simulink model "boolCheck"  (R2022b)
settings: Solver=VariableStepAuto  StartTime=0.0  StopTime=10.0  RelTol=1e-3
settings Model: Creator=ChrisGeorge  LastModifiedBy=ChrisGeorge

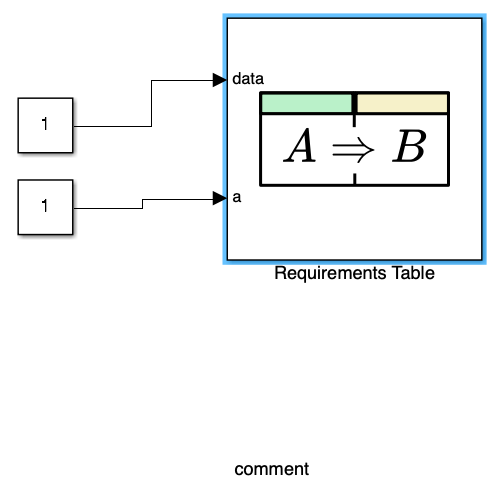
[thumbnail: Simulink's stored preview of the top-level diagram]
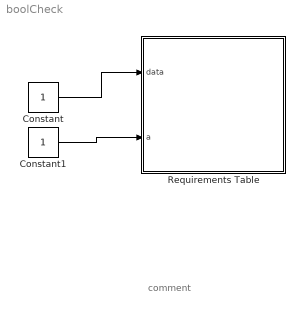
== system boolCheck ==
  note: comment
  Constant : Constant
  Constant1 : Constant
  Requirements Table : Requirements Table  TreatAsAtomicUnit=on
  wires:
  Constant/1 -> Requirements Table/1(data)
  Constant1/1 -> Requirements Table/2(a)

== stateflow chart boolCheck/Requirements Table ==
  (default) -> (junction 1073741860)
  (junction 1073741860) -> (junction 1073741861) : {
      | % SF_REQ_REV_07
      | }
  (junction 1073741861) -> (junction 1073741863) : {
      | % HEADER_ASSIGNMENTS
      |
      | }
  (junction 1073741863) -> (junction 1073741865) : {
      | % START_A_4
      | }
  (junction 1073741865) -> (junction 1073741867) : {
      | }
  (junction 1073741867) -> (junction 1073741869)
  (junction 1073741869) -> (junction 1073741871) : {
      | }
  (junction 1073741871) -> (junction 1073741873) : {
      | % END_A_4
      | }
  (junction 1073741873) -> (junction 1073741911) : {
      | % START_R_1
      | }
  (junction 1073741911) -> (junction 1073741913) : {
      | }
  (junction 1073741913) -> (junction 1073741915)
  (junction 1073741915) -> (junction 1073741917) [order 1] : [((data < 10) | (data > 10) & (data  > 10))]
  (junction 1073741915) -> (junction 1073741923) [order 2]
  (junction 1073741917) -> (junction 1073741919) : {
      | reqtable_postcondition((a > 0), 'R:1');
      |
      |
      | }
  (junction 1073741919) -> (junction 1073741921) : {
      | }
  (junction 1073741921) -> (junction 1073741923)
  (junction 1073741923) -> (junction 1073741925)
  (junction 1073741925) -> (junction 1073741927) : {
      | % END_R_1
      | }
  (junction 1073741927) -> (junction 1073741945) : {
      | % START_R_7
      | }
  (junction 1073741945) -> (junction 1073741947) : {
      | }
  (junction 1073741947) -> (junction 1073741949)
  (junction 1073741949) -> (junction 1073741951) [order 1] : [((data < 10) | (data > 10) && (data  > 10))]
  (junction 1073741949) -> (junction 1073741957) [order 2]
  (junction 1073741951) -> (junction 1073741953) : {
      | reqtable_postcondition((a > 0), 'R:2');
      |
      |
      | }
  (junction 1073741953) -> (junction 1073741955) : {
      | }
  (junction 1073741955) -> (junction 1073741957)
  (junction 1073741957) -> (junction 1073741959)
  (junction 1073741959) -> (junction 1073741961) : {
      | % END_R_7
      | }
  data: data input; a input
